simulink model "Power_Grid_Fault_Analysis_2016"  (R2016a)
settings: Solver=FixedStepAuto  SolverMode=SingleTasking  StartTime=0.0  StopTime=0.2  RelTol=1e-3
InitFcn:
  | basekV = 23;
  | baseMVA = 100;
  | 
  | % base impedance
  | baseZ = (basekV)^2/baseMVA;
  | 
  | % nominal frequency
  | freq = 50;
libraries: powerlib x64, powerlib_meascontrol x17
(part 1 of 4)
settings Model: Creator=jywon  LastModifiedBy=md ether
settings DebuggingCC: SFUnexpectedBacktrackingDiag=error  SFNoUnconditionalDefaultTransitionDiag=error
settings SFSimCC: SimUseLocalCustomCode=on
settings RTWCC: RTWUseLocalCustomCode=on
settings GRTTargetCC: TargetLangStandard=C99 (ISO)  GeneratePreprocessorConditionals=Use local settings
settings ConfigComp: CovMetricSettings=dwe  CovHtmlReporting=off  CovSaveCumulativeToWorkspaceVar=off  CovSaveSingleToWorkspaceVar=off  CovExternalEMLEnable=on

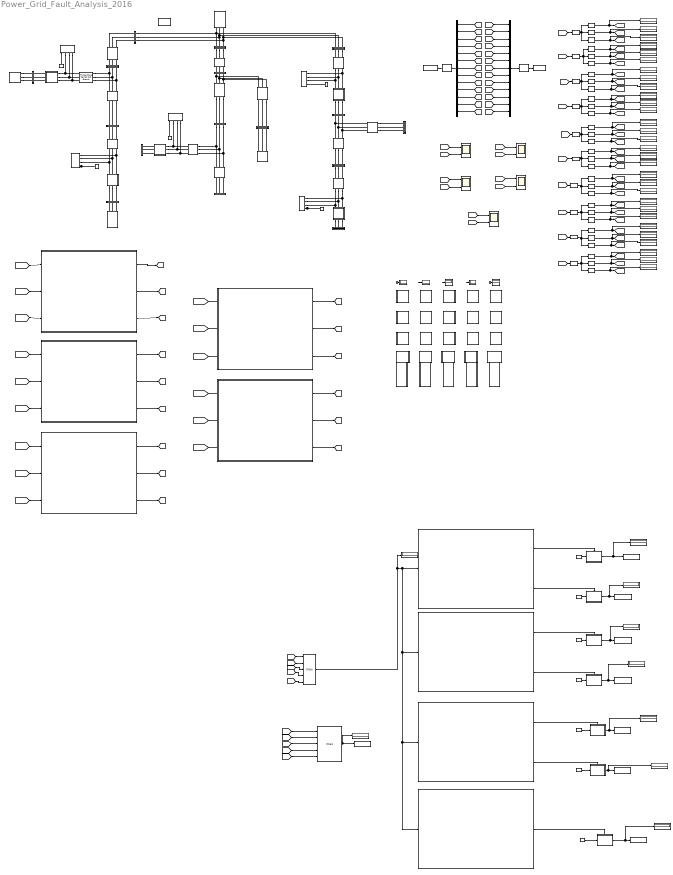
== system Power_Grid_Fault_Analysis_2016 ==
  note: Km S
  note: Fault Phase Detection
  note: Phase Splitter
  note: Zone 1
  note: Zone Voltage and Current
  note: Zone 1
  note: IEEE 16 Bus System
  note: Output Voltage & Current
  note: Zone 2
  note: Zone 5
  note: Zone 4
  note: Zone 3
  note: Zone 1
  note: Zone 2
  note: Zone 3
  note: Zone 4
  note: Zone 5
  note: Zone 2
  note: Zone 3
  note: Zone 4
  note: Zone 5
  note: Km WS
  note: Km S
  note: Km E
  note: Km SE
  Branch1-4 : powerlib/Elements/Three-Phase Series RLC Branch  LConnTagsString=A|B|C  RConnTagsString=A|B|C  BranchType=RL  Resistance=0.075*baseZ  Inductance=(0.1*baseZ)/(2*pi*freq)  Capacitance=1e-6  Measurements=None
  Branch13-14 : powerlib/Elements/Three-Phase Series RLC Branch  LConnTagsString=A|B|C  RConnTagsString=A|B|C  BranchType=RL  Resistance=0.09*baseZ  Inductance=(0.12*baseZ)/(2*pi*freq)  Capacitance=1e-6  Measurements=None
  Branch13-15 : powerlib/Elements/Three-Phase Series RLC Branch  LConnTagsString=A|B|C  RConnTagsString=A|B|C  BranchType=RL  Resistance=0.08*baseZ  Inductance=(0.11*baseZ)/(2*pi*freq)  Capacitance=1e-6  Measurements=None
  Branch15-16 : powerlib/Elements/Three-Phase Series RLC Branch  LConnTagsString=A|B|C  RConnTagsString=A|B|C  BranchType=RL  Resistance=0.04*baseZ  Inductance=(0.04*baseZ)/(2*pi*freq)  Capacitance=1e-6  Measurements=None
  Branch2-8 : powerlib/Elements/Three-Phase Series RLC Branch  LConnTagsString=A|B|C  RConnTagsString=A|B|C  BranchType=RL  Resistance=0.11*baseZ  Inductance=(0.11*baseZ)/(2*pi*freq)  Capacitance=1e-6  Measurements=None
  Branch3-13 : powerlib/Elements/Three-Phase Series RLC Branch  LConnTagsString=A|B|C  RConnTagsString=A|B|C  BranchType=RL  Resistance=0.11*baseZ  Inductance=(0.11*baseZ)/(2*pi*freq)  Capacitance=1e-6  Measurements=None
  Branch4-5 : powerlib/Elements/Three-Phase Series RLC Branch  LConnTagsString=A|B|C  RConnTagsString=A|B|C  BranchType=RL  Resistance=0.08*baseZ  Inductance=(0.11*baseZ)/(2*pi*freq)  Capacitance=1e-6  Measurements=None
  Branch4-6 : powerlib/Elements/Three-Phase Series RLC Branch  LConnTagsString=A|B|C  RConnTagsString=A|B|C  BranchType=RL  Resistance=0.09*baseZ  Inductance=(0.18*baseZ)/(2*pi*freq)  Capacitance=1e-6  Measurements=None
  Branch6-7 : powerlib/Elements/Three-Phase Series RLC Branch  LConnTagsString=A|B|C  RConnTagsString=A|B|C  BranchType=RL  Resistance=0.04  Inductance=(0.04*baseZ)/(2*pi*freq)  Capacitance=1e-6  Measurements=None
  Branch8-10 : powerlib/Elements/Three-Phase Series RLC Branch  LConnTagsString=A|B|C  RConnTagsString=A|B|C  BranchType=RL  Resistance=0.11*baseZ  Inductance=(0.11*baseZ)/(2*pi*freq)  Capacitance=1e-6  Measurements=None
  Branch8-9 : powerlib/Elements/Three-Phase Series RLC Branch  LConnTagsString=A|B|C  RConnTagsString=A|B|C  BranchType=RL  Resistance=0.08*baseZ  Inductance=(0.11*baseZ)/(2*pi*freq)  Capacitance=1e-6  Measurements=None
  Branch9-11 : powerlib/Elements/Three-Phase Series RLC Branch  LConnTagsString=A|B|C  RConnTagsString=A|B|C  BranchType=RL  Resistance=0.11*baseZ  Inductance=(0.11*baseZ)/(2*pi*freq)  Capacitance=1e-6  Measurements=None
  Branch9-12 : powerlib/Elements/Three-Phase Series RLC Branch  LConnTagsString=A|B|C  RConnTagsString=A|B|C  BranchType=RL  Resistance=0.08*baseZ  Inductance=(0.11*baseZ)/(2*pi*freq)  Capacitance=1e-6  Measurements=None
  Bus_1 : Subsystem
  Bus_10 : Subsystem
  Bus_11 : Subsystem
  Bus_12 : Subsystem
  Bus_13 : Subsystem
  Bus_14 : Subsystem
  Bus_15 : Subsystem
  Bus_16 : Subsystem
  Bus_2 : Subsystem
  Bus_3 : Subsystem
  Bus_4 : Subsystem
  Bus_5 : Subsystem
  Bus_6 : Subsystem
  Bus_7 : Subsystem
  Bus_8 : Subsystem
  Bus_9 : Subsystem
  Constant{,1..2,4} (4 alike) : Constant  Value=0
  Constant10 : Constant  Value=5
  Constant11 : Constant  Value=7
  Constant3 : Constant
  Constant5 : Constant  Value=2
  Constant6 : Constant  Value=4
  Constant7 : Constant  Value=3
  Constant8 : Constant
  Constant9 : Constant  Value=6
  Display{,1..43} (44 alike) : Display
      Display settings: Decimation=2
      Display1 settings: Decimation=2
      Display10 settings: Decimation=2
      Display11 settings: Decimation=2
      Display12 settings: Decimation=2
      Display13 settings: Decimation=2
      Display14 settings: Decimation=2
      Display15 settings: Decimation=2
      Display16 settings: Decimation=2
      Display17 settings: Decimation=2
      Display18 settings: Decimation=2
      Display19 settings: Decimation=2
      Display2 settings: Decimation=2
      Display20 settings: Decimation=2
      Display21 settings: Decimation=2
      Display22 settings: Decimation=2
      Display23 settings: Decimation=2
      Display24 settings: Decimation=2
      Display25 settings: Decimation=2
      Display26 settings: Decimation=2
      Display27 settings: Decimation=2
      Display28 settings: Decimation=2
      Display29 settings: Decimation=2
      Display3 settings: Decimation=2
      Display4 settings: Decimation=2
      Display5 settings: Decimation=2
      Display6 settings: Decimation=2
      Display7 settings: Decimation=2
      Display8 settings: Decimation=2
      Display9 settings: Decimation=2
  For Zone 1 : Subsystem
  For Zone 2 : Subsystem
  For Zone 3 : Subsystem
  For Zone 4 : Subsystem
  For Zone 5 : Subsystem
  If : If  IfExpression=u1==1|u1==8|u1==15|u1==22|u1==29  ElseIfExpressions=u1==2|u1==9|u1==16|u1==23|u1==30  ShowElse=off
  If Action Subsystem : Subsystem  TreatAsAtomicUnit=on
  If Action Subsystem1 : Subsystem  TreatAsAtomicUnit=on
  If Action Subsystem2 : Subsystem  TreatAsAtomicUnit=on
  If Action Subsystem3 : Subsystem  TreatAsAtomicUnit=on
  If Action Subsystem4 : Subsystem  TreatAsAtomicUnit=on
  If Action Subsystem5 : Subsystem  TreatAsAtomicUnit=on
  If Action Subsystem6 : Subsystem  TreatAsAtomicUnit=on
  If1 : If  IfExpression=u1==3|u1==10|u1==17|u1==24|u1==31  ElseIfExpressions=u1==4|u1==11|u1==18|u1==25|u1==32  ShowElse=off
  If2 : If  IfExpression=u1==5|u1==12|u1==19|u1==26|u1==33  ElseIfExpressions=u1==6|u1==13|u1==20|u1==27|u1==34  ShowElse=off
  If3 : If  IfExpression=u1==7|u1==14|u1==21|u1==28|u1==35  ShowElse=off
  Incoming1 : powerlib/Electrical Sources/Three-Phase Source  InternalConnection=Yg  VoltagePhases=off  Voltage=basekV*1e3  PhaseAngle=0  Voltage_phases=[25e3 25e3 25e3]/sqrt(3)  PhaseAngles_phases=[0 -120 +120]  Frequency=freq  NonIdealSource=off  SpecifyImpedance=on  Resistance=0.8929  Inductance=16.58e-3  ShortCircuitLevel=438.555e6  BaseVoltage=12.66e3  XRratio=7  BusType=swing  Pref=0  Qref=0  Prefabc=[10e3, 10e3, 10e3]  Qrefabc=[0, 0, 0]  Qmin=-inf  Qmax=inf
  Lamp1 : Subsystem  DialogController=hmiCreateDDGDialog  IsWebBlock=on  mask(MWDashboardBlock){webBlockId=468f77b7-8d3f-43ba-abb4-7f9de16ce9e1, webBlockType=lamp, ShowInLibBrowser=on, ShowInitialText=on, HMISrcModelName=Power_Grid_Fault_Analysis_2016}
      mask prompts: webBlockId "WebBlock Id"; webBlockType "WebBlock Type"; HMISrcModelName "Source Model"
      mask help: Display a color that reflects an input value.
      mask Help: helpview([docroot '/mapfiles/simulink.map'], 'hmi_lamp')
      mask Display:
      | if strcmp(get_param(bdroot(gcb),'BlockDiagramType'),'library')
      |  image([(matlabroot) '/toolbox/simulink/hmi/icons/Lamp.png'])
      | end
  Lamp10 : Subsystem  DialogController=hmiCreateDDGDialog  IsWebBlock=on  mask(MWDashboardBlock){webBlockId=47d835ee-9e52-457b-b3a4-dabcf9efd005, webBlockType=lamp, ShowInLibBrowser=on, ShowInitialText=on, HMISrcModelName=Power_Grid_Fault_Analysis_2016}
      mask prompts: webBlockId "WebBlock Id"; webBlockType "WebBlock Type"; HMISrcModelName "Source Model"
      mask help: Display a color that reflects an input value.
      mask Help: helpview([docroot '/mapfiles/simulink.map'], 'hmi_lamp')
      mask Display:
      | if strcmp(get_param(bdroot(gcb),'BlockDiagramType'),'library')
      |  image([(matlabroot) '/toolbox/simulink/hmi/icons/Lamp.png'])
      | end
  Lamp11 : Subsystem  DialogController=hmiCreateDDGDialog  IsWebBlock=on  mask(MWDashboardBlock){webBlockId=f8b1e46b-6cbe-4fd8-a06e-1cc90b8c3338, webBlockType=lamp, ShowInLibBrowser=on, ShowInitialText=on, HMISrcModelName=Power_Grid_Fault_Analysis_2016}
      mask prompts: webBlockId "WebBlock Id"; webBlockType "WebBlock Type"; HMISrcModelName "Source Model"
      mask help: Display a color that reflects an input value.
      mask Help: helpview([docroot '/mapfiles/simulink.map'], 'hmi_lamp')
      mask Display:
      | if strcmp(get_param(bdroot(gcb),'BlockDiagramType'),'library')
      |  image([(matlabroot) '/toolbox/simulink/hmi/icons/Lamp.png'])
      | end
  Lamp12 : Subsystem  DialogController=hmiCreateDDGDialog  IsWebBlock=on  mask(MWDashboardBlock){webBlockId=2111019f-f01e-48a9-874b-3a281ad1a610, webBlockType=lamp, ShowInLibBrowser=on, ShowInitialText=on, HMISrcModelName=Power_Grid_Fault_Analysis_2016}
      mask prompts: webBlockId "WebBlock Id"; webBlockType "WebBlock Type"; HMISrcModelName "Source Model"
      mask help: Display a color that reflects an input value.
      mask Help: helpview([docroot '/mapfiles/simulink.map'], 'hmi_lamp')
      mask Display:
      | if strcmp(get_param(bdroot(gcb),'BlockDiagramType'),'library')
      |  image([(matlabroot) '/toolbox/simulink/hmi/icons/Lamp.png'])
      | end
  Lamp14 : Subsystem  DialogController=hmiCreateDDGDialog  IsWebBlock=on  mask(MWDashboardBlock){webBlockId=0497d169-c07f-488b-b667-ee60b9bfb21c, webBlockType=lamp, ShowInLibBrowser=on, ShowInitialText=on, HMISrcModelName=Power_Grid_Fault_Analysis_2016}
      mask prompts: webBlockId "WebBlock Id"; webBlockType "WebBlock Type"; HMISrcModelName "Source Model"
      mask help: Display a color that reflects an input value.
      mask Help: helpview([docroot '/mapfiles/simulink.map'], 'hmi_lamp')
      mask Display:
      | if strcmp(get_param(bdroot(gcb),'BlockDiagramType'),'library')
      |  image([(matlabroot) '/toolbox/simulink/hmi/icons/Lamp.png'])
      | end
  Lamp15 : Subsystem  DialogController=hmiCreateDDGDialog  IsWebBlock=on  mask(MWDashboardBlock){webBlockId=37fb807e-8b4a-4eb5-8cd1-eaf9de247767, webBlockType=lamp, ShowInLibBrowser=on, ShowInitialText=on, HMISrcModelName=Power_Grid_Fault_Analysis_2016}
      mask prompts: webBlockId "WebBlock Id"; webBlockType "WebBlock Type"; HMISrcModelName "Source Model"
      mask help: Display a color that reflects an input value.
      mask Help: helpview([docroot '/mapfiles/simulink.map'], 'hmi_lamp')
      mask Display:
      | if strcmp(get_param(bdroot(gcb),'BlockDiagramType'),'library')
      |  image([(matlabroot) '/toolbox/simulink/hmi/icons/Lamp.png'])
      | end
  Lamp16 : Subsystem  DialogController=hmiCreateDDGDialog  IsWebBlock=on  mask(MWDashboardBlock){webBlockId=dff293cc-569e-47d8-a4fe-e96dd9d4666d, webBlockType=lamp, ShowInLibBrowser=on, ShowInitialText=on, HMISrcModelName=Power_Grid_Fault_Analysis_2016}
      mask prompts: webBlockId "WebBlock Id"; webBlockType "WebBlock Type"; HMISrcModelName "Source Model"
      mask help: Display a color that reflects an input value.
      mask Help: helpview([docroot '/mapfiles/simulink.map'], 'hmi_lamp')
      mask Display:
      | if strcmp(get_param(bdroot(gcb),'BlockDiagramType'),'library')
      |  image([(matlabroot) '/toolbox/simulink/hmi/icons/Lamp.png'])
      | end
  Lamp18 : Subsystem  DialogController=hmiCreateDDGDialog  IsWebBlock=on  mask(MWDashboardBlock){webBlockId=13b1519a-e014-4802-8a4a-79357282a9e7, webBlockType=lamp, ShowInLibBrowser=on, ShowInitialText=on, HMISrcModelName=Power_Grid_Fault_Analysis_2016}
      mask prompts: webBlockId "WebBlock Id"; webBlockType "WebBlock Type"; HMISrcModelName "Source Model"
      mask help: Display a color that reflects an input value.
      mask Help: helpview([docroot '/mapfiles/simulink.map'], 'hmi_lamp')
      mask Display:
      | if strcmp(get_param(bdroot(gcb),'BlockDiagramType'),'library')
      |  image([(matlabroot) '/toolbox/simulink/hmi/icons/Lamp.png'])
      | end
  Lamp19 : Subsystem  DialogController=hmiCreateDDGDialog  IsWebBlock=on  mask(MWDashboardBlock){webBlockId=26516c08-3b96-4d03-8fdb-bfe990d7f45b, webBlockType=lamp, ShowInLibBrowser=on, ShowInitialText=on, HMISrcModelName=Power_Grid_Fault_Analysis_2016}
      mask prompts: webBlockId "WebBlock Id"; webBlockType "WebBlock Type"; HMISrcModelName "Source Model"
      mask help: Display a color that reflects an input value.
      mask Help: helpview([docroot '/mapfiles/simulink.map'], 'hmi_lamp')
      mask Display:
      | if strcmp(get_param(bdroot(gcb),'BlockDiagramType'),'library')
      |  image([(matlabroot) '/toolbox/simulink/hmi/icons/Lamp.png'])
      | end
  Lamp2 : Subsystem  DialogController=hmiCreateDDGDialog  IsWebBlock=on  mask(MWDashboardBlock){webBlockId=3d3c35ee-dc2a-417a-bf5a-5478148348c2, webBlockType=lamp, ShowInLibBrowser=on, ShowInitialText=on, HMISrcModelName=Power_Grid_Fault_Analysis_2016}
      mask prompts: webBlockId "WebBlock Id"; webBlockType "WebBlock Type"; HMISrcModelName "Source Model"
      mask help: Display a color that reflects an input value.
      mask Help: helpview([docroot '/mapfiles/simulink.map'], 'hmi_lamp')
      mask Display:
      | if strcmp(get_param(bdroot(gcb),'BlockDiagramType'),'library')
      |  image([(matlabroot) '/toolbox/simulink/hmi/icons/Lamp.png'])
      | end
  Lamp20 : Subsystem  DialogController=hmiCreateDDGDialog  IsWebBlock=on  mask(MWDashboardBlock){webBlockId=6f7fce04-8c20-4fba-bd33-a90a1905ab0b, webBlockType=lamp, ShowInLibBrowser=on, ShowInitialText=on, HMISrcModelName=Power_Grid_Fault_Analysis_2016}
      mask prompts: webBlockId "WebBlock Id"; webBlockType "WebBlock Type"; HMISrcModelName "Source Model"
      mask help: Display a color that reflects an input value.
      mask Help: helpview([docroot '/mapfiles/simulink.map'], 'hmi_lamp')
      mask Display:
      | if strcmp(get_param(bdroot(gcb),'BlockDiagramType'),'library')
      |  image([(matlabroot) '/toolbox/simulink/hmi/icons/Lamp.png'])
      | end
  Lamp21 : Subsystem  DialogController=hmiCreateDDGDialog  IsWebBlock=on  mask(MWDashboardBlock){webBlockId=c64cc1d0-1ee1-41b0-b1ef-29387c8c4faf, webBlockType=lamp, ShowInLibBrowser=on, ShowInitialText=on, HMISrcModelName=Power_Grid_Fault_Analysis_2016}
      mask prompts: webBlockId "WebBlock Id"; webBlockType "WebBlock Type"; HMISrcModelName "Source Model"
      mask help: Display a color that reflects an input value.
      mask Help: helpview([docroot '/mapfiles/simulink.map'], 'hmi_lamp')
      mask Display:
      | if strcmp(get_param(bdroot(gcb),'BlockDiagramType'),'library')
      |  image([(matlabroot) '/toolbox/simulink/hmi/icons/Lamp.png'])
      | end
  Lamp22 : Subsystem  DialogController=hmiCreateDDGDialog  IsWebBlock=on  mask(MWDashboardBlock){webBlockId=845159ea-2f47-481f-a3ef-47166ce66799, webBlockType=lamp, ShowInLibBrowser=on, ShowInitialText=on, HMISrcModelName=Power_Grid_Fault_Analysis_2016}
      mask prompts: webBlockId "WebBlock Id"; webBlockType "WebBlock Type"; HMISrcModelName "Source Model"
      mask help: Display a color that reflects an input value.
      mask Help: helpview([docroot '/mapfiles/simulink.map'], 'hmi_lamp')
      mask Display:
      | if strcmp(get_param(bdroot(gcb),'BlockDiagramType'),'library')
      |  image([(matlabroot) '/toolbox/simulink/hmi/icons/Lamp.png'])
      | end
  Lamp23 : Subsystem  DialogController=hmiCreateDDGDialog  IsWebBlock=on  mask(MWDashboardBlock){webBlockId=af2698c2-590e-4ed0-a645-40a46a76e42b, webBlockType=lamp, ShowInLibBrowser=on, ShowInitialText=on, HMISrcModelName=Power_Grid_Fault_Analysis_2016}
      mask prompts: webBlockId "WebBlock Id"; webBlockType "WebBlock Type"; HMISrcModelName "Source Model"
      mask help: Display a color that reflects an input value.
      mask Help: helpview([docroot '/mapfiles/simulink.map'], 'hmi_lamp')
      mask Display:
      | if strcmp(get_param(bdroot(gcb),'BlockDiagramType'),'library')
      |  image([(matlabroot) '/toolbox/simulink/hmi/icons/Lamp.png'])
      | end
  Lamp3 : Subsystem  DialogController=hmiCreateDDGDialog  IsWebBlock=on  mask(MWDashboardBlock){webBlockId=b3a08374-8d73-4b38-9446-1522d8dad8a0, webBlockType=lamp, ShowInLibBrowser=on, ShowInitialText=on, HMISrcModelName=Power_Grid_Fault_Analysis_2016}
      mask prompts: webBlockId "WebBlock Id"; webBlockType "WebBlock Type"; HMISrcModelName "Source Model"
      mask help: Display a color that reflects an input value.
      mask Help: helpview([docroot '/mapfiles/simulink.map'], 'hmi_lamp')
      mask Display:
      | if strcmp(get_param(bdroot(gcb),'BlockDiagramType'),'library')
      |  image([(matlabroot) '/toolbox/simulink/hmi/icons/Lamp.png'])
      | end
  Lamp4 : Subsystem  DialogController=hmiCreateDDGDialog  IsWebBlock=on  mask(MWDashboardBlock){webBlockId=b5af589e-626e-4b25-93a4-676fcf5d279b, webBlockType=lamp, ShowInLibBrowser=on, ShowInitialText=on, HMISrcModelName=Power_Grid_Fault_Analysis_2016}
      mask prompts: webBlockId "WebBlock Id"; webBlockType "WebBlock Type"; HMISrcModelName "Source Model"
      mask help: Display a color that reflects an input value.
      mask Help: helpview([docroot '/mapfiles/simulink.map'], 'hmi_lamp')
      mask Display:
      | if strcmp(get_param(bdroot(gcb),'BlockDiagramType'),'library')
      |  image([(matlabroot) '/toolbox/simulink/hmi/icons/Lamp.png'])
      | end
  Lamp5 : Subsystem  DialogController=hmiCreateDDGDialog  IsWebBlock=on  mask(MWDashboardBlock){webBlockId=8c5f1737-98a7-4483-befe-b85a709fdb78, webBlockType=lamp, ShowInLibBrowser=on, ShowInitialText=on, HMISrcModelName=Power_Grid_Fault_Analysis_2016}
      mask prompts: webBlockId "WebBlock Id"; webBlockType "WebBlock Type"; HMISrcModelName "Source Model"
      mask help: Display a color that reflects an input value.
      mask Help: helpview([docroot '/mapfiles/simulink.map'], 'hmi_lamp')
      mask Display:
      | if strcmp(get_param(bdroot(gcb),'BlockDiagramType'),'library')
      |  image([(matlabroot) '/toolbox/simulink/hmi/icons/Lamp.png'])
      | end
  Lamp6 : Subsystem  DialogController=hmiCreateDDGDialog  IsWebBlock=on  mask(MWDashboardBlock){webBlockId=54263707-eb2a-444c-8d6c-36b23799e939, webBlockType=lamp, ShowInLibBrowser=on, ShowInitialText=on, HMISrcModelName=Power_Grid_Fault_Analysis_2016}
      mask prompts: webBlockId "WebBlock Id"; webBlockType "WebBlock Type"; HMISrcModelName "Source Model"
      mask help: Display a color that reflects an input value.
      mask Help: helpview([docroot '/mapfiles/simulink.map'], 'hmi_lamp')
      mask Display:
      | if strcmp(get_param(bdroot(gcb),'BlockDiagramType'),'library')
      |  image([(matlabroot) '/toolbox/simulink/hmi/icons/Lamp.png'])
      | end
  Lamp7 : Subsystem  DialogController=hmiCreateDDGDialog  IsWebBlock=on  mask(MWDashboardBlock){webBlockId=44ba34c8-8d6e-4af3-8262-8e210390e885, webBlockType=lamp, ShowInLibBrowser=on, ShowInitialText=on, HMISrcModelName=Power_Grid_Fault_Analysis_2016}
      mask prompts: webBlockId "WebBlock Id"; webBlockType "WebBlock Type"; HMISrcModelName "Source Model"
      mask help: Display a color that reflects an input value.
      mask Help: helpview([docroot '/mapfiles/simulink.map'], 'hmi_lamp')
      mask Display:
      | if strcmp(get_param(bdroot(gcb),'BlockDiagramType'),'library')
      |  image([(matlabroot) '/toolbox/simulink/hmi/icons/Lamp.png'])
      | end
  Lamp9 : Subsystem  DialogController=hmiCreateDDGDialog  IsWebBlock=on  mask(MWDashboardBlock){webBlockId=ca856779-7c2c-42aa-8051-6cc6fb4e4d11, webBlockType=lamp, ShowInLibBrowser=on, ShowInitialText=on, HMISrcModelName=Power_Grid_Fault_Analysis_2016}
      mask prompts: webBlockId "WebBlock Id"; webBlockType "WebBlock Type"; HMISrcModelName "Source Model"
      mask help: Display a color that reflects an input value.
      mask Help: helpview([docroot '/mapfiles/simulink.map'], 'hmi_lamp')
      mask Display:
      | if strcmp(get_param(bdroot(gcb),'BlockDiagramType'),'library')
      |  image([(matlabroot) '/toolbox/simulink/hmi/icons/Lamp.png'])
      | end
  Max : MinMax  Function=max  Inputs=5
  Max1 : MinMax  Function=max  Inputs=5
  Mux : Mux  Inputs=13
  Mux1 : Mux  Inputs=13
  RMS{,1..11} (12 alike) : powerlib_meascontrol/Measurements/RMS  TrueRMS=on  Freq=freq  RMSInit=0  Ts=0
  "Relay " : Subsystem
  Relay 1 : Subsystem
  Relay 2 : Subsystem
  Relay 3 : Subsystem
  Relay 4 : Subsystem
  Scope{,1..4} (5 alike) : Scope  NumInputPorts=2
  Selector{,3,6,9,14,17,20,23,26,29} (10 alike) : Selector  InputPortWidth=3  IndexOptions=Index vector (dialog)  Indices=[1]  OutputSizes=1
  Selector{1,4,7,10,12,15,18,21,24,27} (10 alike) : Selector  InputPortWidth=3  IndexOptions=Index vector (dialog)  Indices=[2]  OutputSizes=1
  Selector{2,5,8,11,13,16,19,22,25,28} (10 alike) : Selector  InputPortWidth=3  IndexOptions=Index vector (dialog)  Indices=[3]  OutputSizes=1
  Three-Phase Fault1 : powerlib/Elements/Three-Phase Fault  InitialStates=[0 0 0]  FaultA=on  FaultB=off  FaultC=off  GroundFault=on  SwitchTimes="[1/60  5/60]"  External=on  SwitchStatus=NaN  FaultResistance=0.1  GroundResistance=0.01  SnubberResistance=1e6  SnubberCapacitance=inf  Measurements=None
  Three-Phase Fault2 : powerlib/Elements/Three-Phase Fault  InitialStates=[0 0 0]  FaultA=on  FaultB=on  FaultC=off  GroundFault=on  SwitchTimes="[1/60  5/60]"  External=on  SwitchStatus=NaN  FaultResistance=0.1  GroundResistance=0.01  SnubberResistance=1e6  SnubberCapacitance=inf  Measurements=None
  Three-Phase Fault3 : powerlib/Elements/Three-Phase Fault  InitialStates=[0 0 0]  FaultA=on  FaultB=on  FaultC=on  GroundFault=on  SwitchTimes="[1/60  5/60]"  External=on  SwitchStatus=NaN  FaultResistance=0.1  GroundResistance=0.01  SnubberResistance=1e6  SnubberCapacitance=inf  Measurements=None
  Three-Phase Fault4 : powerlib/Elements/Three-Phase Fault  InitialStates=[0 0 0]  FaultA=on  FaultB=off  FaultC=off  GroundFault=on  SwitchTimes="[1/60  5/60]"  External=on  SwitchStatus=NaN  FaultResistance=0.1  GroundResistance=0.01  SnubberResistance=1e6  SnubberCapacitance=inf  Measurements=None
  Three-Phase Fault5 : powerlib/Elements/Three-Phase Fault  InitialStates=[0 0 0]  FaultA=on  FaultB=off  FaultC=off  GroundFault=on  SwitchTimes="[1/60  5/60]"  External=on  SwitchStatus=NaN  FaultResistance=0.1  GroundResistance=0.01  SnubberResistance=1e6  SnubberCapacitance=inf  Measurements=None
  Tieline10-14 : powerlib/Elements/Three-Phase Series RLC Branch  LConnTagsString=A|B|C  RConnTagsString=A|B|C  BranchType=RL  Resistance=0.04*baseZ  Inductance=(0.04*baseZ)/(2*pi*freq)  Capacitance=1e-6  Measurements=None
  Tieline5-11 : powerlib/Elements/Three-Phase Series RLC Branch  LConnTagsString=A|B|C  RConnTagsString=A|B|C  BranchType=RL  Resistance=0.04*baseZ  Inductance=(0.04*baseZ)/(2*pi*freq)  Capacitance=1e-6  Measurements=None
  Tieline7-16 : powerlib/Elements/Three-Phase Series RLC Branch  LConnTagsString=A|B|C  RConnTagsString=A|B|C  BranchType=RL  Resistance=0.09*baseZ  Inductance=(0.12*baseZ)/(2*pi*freq)  Capacitance=1e-6  Measurements=None
  To Workspace : ToWorkspace  VariableName=simOutputV  SaveFormat=Timeseries  SampleTime=-1
  To Workspace1 : ToWorkspace  VariableName=simOutputI  SaveFormat=Timeseries  SampleTime=-1
  To Workspace2 : ToWorkspace  VariableName=Distance  SaveFormat=Timeseries  SampleTime=-1
  To Workspace3 : ToWorkspace  VariableName=A  SaveFormat=Timeseries  SampleTime=-1
  To Workspace4 : ToWorkspace  VariableName=B  SaveFormat=Timeseries  SampleTime=-1
  To Workspace5 : ToWorkspace  VariableName=C  SaveFormat=Timeseries  SampleTime=-1
  To Workspace6 : ToWorkspace  VariableName=AB  SaveFormat=Timeseries  SampleTime=-1
  To Workspace7 : ToWorkspace  VariableName=BC  SaveFormat=Timeseries  SampleTime=-1
  To Workspace8 : ToWorkspace  VariableName=CA  SaveFormat=Timeseries  SampleTime=-1
  To Workspace9 : ToWorkspace  VariableName=ABC  SaveFormat=Timeseries  SampleTime=-1
  Toggle Switch : Subsystem  DialogController=hmiCreateDDGDialog  IsWebBlock=on  mask(MWDashboardBlock){webBlockId=0d8ce81f-dbe4-4348-a7f3-529ab13bc594, webBlockType=toggleswitch, ShowInLibBrowser=on, ShowInitialText=on, HMISrcModelName=Power_Grid_Fault_Analysis_2016}
      mask prompts: webBlockId "WebBlock Id"; webBlockType "WebBlock Type"; HMISrcModelName "Source Model"
      mask help: Set on/off value to tune parameters or variables.
      mask Help: helpview([docroot '/mapfiles/simulink.map'], 'hmi_switch')
      mask Display:
      | if strcmp(get_param(bdroot(gcb),'BlockDiagramType'),'library')
      |  image([(matlabroot) '/toolbox/simulink/hmi/icons/ToggleSwitch.png'])
      | end
  Toggle Switch1 : Subsystem  DialogController=hmiCreateDDGDialog  IsWebBlock=on  mask(MWDashboardBlock){webBlockId=5b9374ce-f1d7-4d86-b5a1-51c8e36ab682, webBlockType=toggleswitch, ShowInLibBrowser=on, ShowInitialText=on, HMISrcModelName=Power_Grid_Fault_Analysis_2016}
      mask prompts: webBlockId "WebBlock Id"; webBlockType "WebBlock Type"; HMISrcModelName "Source Model"
      mask help: Set on/off value to tune parameters or variables.
      mask Help: helpview([docroot '/mapfiles/simulink.map'], 'hmi_switch')
      mask Display:
      | if strcmp(get_param(bdroot(gcb),'BlockDiagramType'),'library')
      |  image([(matlabroot) '/toolbox/simulink/hmi/icons/ToggleSwitch.png'])
      | end
  Toggle Switch2 : Subsystem  DialogController=hmiCreateDDGDialog  IsWebBlock=on  mask(MWDashboardBlock){webBlockId=a5a22a72-9f9a-45fa-8f0f-c647fe18b1da, webBlockType=toggleswitch, ShowInLibBrowser=on, ShowInitialText=on, HMISrcModelName=Power_Grid_Fault_Analysis_2016}
      mask prompts: webBlockId "WebBlock Id"; webBlockType "WebBlock Type"; HMISrcModelName "Source Model"
      mask help: Set on/off value to tune parameters or variables.
      mask Help: helpview([docroot '/mapfiles/simulink.map'], 'hmi_switch')
      mask Display:
      | if strcmp(get_param(bdroot(gcb),'BlockDiagramType'),'library')
      |  image([(matlabroot) '/toolbox/simulink/hmi/icons/ToggleSwitch.png'])
      | end
  Toggle Switch3 : Subsystem  DialogController=hmiCreateDDGDialog  IsWebBlock=on  mask(MWDashboardBlock){webBlockId=58ae28e7-e799-496d-825d-186d552e1de1, webBlockType=toggleswitch, ShowInLibBrowser=on, ShowInitialText=on, HMISrcModelName=Power_Grid_Fault_Analysis_2016}
      mask prompts: webBlockId "WebBlock Id"; webBlockType "WebBlock Type"; HMISrcModelName "Source Model"
      mask help: Set on/off value to tune parameters or variables.
      mask Help: helpview([docroot '/mapfiles/simulink.map'], 'hmi_switch')
      mask Display:
      | if strcmp(get_param(bdroot(gcb),'BlockDiagramType'),'library')
      |  image([(matlabroot) '/toolbox/simulink/hmi/icons/ToggleSwitch.png'])
      | end
  Toggle Switch4 : Subsystem  DialogController=hmiCreateDDGDialog  IsWebBlock=on  mask(MWDashboardBlock){webBlockId=0e496b9f-e035-48d9-ae06-0f0cf0e7b1be, webBlockType=toggleswitch, ShowInLibBrowser=on, ShowInitialText=on, HMISrcModelName=Power_Grid_Fault_Analysis_2016}
      mask prompts: webBlockId "WebBlock Id"; webBlockType "WebBlock Type"; HMISrcModelName "Source Model"
      mask help: Set on/off value to tune parameters or variables.
      mask Help: helpview([docroot '/mapfiles/simulink.map'], 'hmi_switch')
      mask Display:
      | if strcmp(get_param(bdroot(gcb),'BlockDiagramType'),'library')
      |  image([(matlabroot) '/toolbox/simulink/hmi/icons/ToggleSwitch.png'])
      | end
  powergui1 : powerlib/powergui  Priority=1  SimulationMode=Discrete  SampleTime=50e-6  frequency=60  Iterations=50  frequencyindice=50  Pbase=100e6  ErrMax=0.0001  UnitsV=kV  UnitsW=MW  buscounter=0  FunctionMessages=off  echomessages=off  EnableUseOfTLC=off  CurrentSourceSwitches=off  DisableSnubberDevices=off  DisableRonSwitches=off  DisableVfSwitches=off  DisplayEquations=off  AutomaticDiscreteSolvers=off  SolverType=Tustin/Backward Euler (TBE)  Interpol=off  ExternalGateDelay=off  methode=off  Ts=100  x0status=blocks  SPID=off  SwTol=0  HookPort=off  NonlinearTolerance=0  nMaxIteration=15  ContinueOnMaxIteration=off  RestoreLinks=warning  ResistiveCurrentMeasurement=off  Frange=[0:2:500]  Ylog=off  Xlog=on  ShowGrid=off  save=off  variable=ZData  structure=0  ZoomFFT=off  StartTime=0.0  cycles=1  DisplayStyle=1  fundamental=60  FreqAxis=off  MaxFrequency=1000  frequencyindicesteady=1  RmsSteady=2  display=off
  tag scope: B_2=global, B_5=global
  wires:
  [V13to15] -> Mux/12
  [V6to7] -> Mux/4
  [V2to8] -> Mux/5
  [V13to14] -> Mux/11
  [V4to6] -> Mux/3
  [V8to9] -> Mux/6
  [V4to5] -> Mux/2
  [V15to16] -> Mux/13
  Mux/1 -> RMS/1
  [V9to11] -> Mux/8
  [V1to4] -> Mux/1
  [V8to10] -> Mux/7
  [V3to13] -> Mux/10
  RMS1/1 -> To Workspace1/1
  RMS/1 -> To Workspace/1
  [V9to12] -> Mux/9
  [I8to9] -> Mux1/6
  [I13to14] -> Mux1/11
  [I6to7] -> Mux1/4
  [I2to8] -> Mux1/5
  [I1to4] -> Mux1/1
  [I4to5] -> Mux1/2
  [I13to15] -> Mux1/12
  [I9to12] -> Mux1/9
  [I3to13] -> Mux1/10
  [I15to16] -> Mux1/13
  [I4to6] -> Mux1/3
  [I9to11] -> Mux1/8
  [I8to10] -> Mux1/7
  Mux1/1 -> RMS1/1
  Constant3/1 -> Three-Phase Fault2/1  "Bus 3-13 Fault"
  [V4to5] -> Scope/1
  [I4to5] -> Scope/2
  Constant4/1 -> [B_5], Three-Phase Fault1/1  "Bus 15-16 Fault"
  Constant2/1 -> Three-Phase Fault3/1  "Bus 9-11 Fault"
  Constant1/1 -> [B_2], Three-Phase Fault4/1  "Bus 6-7 Fault"
  Constant/1 -> Three-Phase Fault5/1  "Z1"
  [I6to7] -> Scope1/2
  [V6to7] -> Scope1/1
  [V3to13] -> Scope3/1
  [I3to13] -> Scope3/2
  [I9to11] -> Scope2/2
  [V9to11] -> Scope2/1
  [I15to16] -> Scope4/2
  [V15to16] -> Scope4/1
  RMS3/1 -> Selector2/1, Selector1/1, Selector/1
  [I4to5] -> RMS2/1
  Selector/1 -> Display/1, [Z1_Va]
  Selector1/1 -> Display1/1, [Z1_Vb]
  Selector2/1 -> Display2/1, [Z1_Vc]
  Selector11/1 -> Display11/1, [Z2_Ic]
  Selector10/1 -> Display10/1, [Z2_Ib]
  Selector9/1 -> Display9/1, [Z2_Ia]
  Selector8/1 -> Display8/1, [Z2_Vc]
  Selector7/1 -> Display7/1, [Z2_Vb]
  Selector6/1 -> Display6/1, [Z2_Va]
  RMS5/1 -> Selector9/1, Selector10/1, Selector11/1
  RMS4/1 -> Selector6/1, Selector7/1, Selector8/1
  Selector13/1 -> Display13/1, [Z3_Ic]
  RMS7/1 -> Selector17/1, Selector12/1, Selector13/1
  Selector15/1 -> Display15/1, [Z3_Vb]
  Selector14/1 -> Display14/1, [Z3_Va]
  RMS6/1 -> Selector14/1, Selector15/1, Selector16/1
  Selector17/1 -> Display17/1, [Z3_Ia]
  Selector12/1 -> Display12/1, [Z3_Ib]
  Selector16/1 -> Display16/1, [Z3_Vc]
  Selector22/1 -> Display22/1, [Z4_Vc]
  Selector18/1 -> Display18/1, [Z4_Ib]
  Selector23/1 -> Display23/1, [Z4_Ia]
  RMS8/1 -> Selector20/1, Selector21/1, Selector22/1
  Selector20/1 -> Display20/1, [Z4_Va]
  Selector21/1 -> Display21/1, [Z4_Vb]
  RMS9/1 -> Selector23/1, Selector18/1, Selector19/1
  Selector19/1 -> Display19/1, [Z4_Ic]
  Selector24/1 -> Display24/1, [Z5_Ib]
  Selector28/1 -> Display28/1, [Z5_Vc]
  RMS10/1 -> Selector26/1, Selector27/1, Selector28/1
  Selector29/1 -> Display29/1, [Z5_Ia]
  Selector25/1 -> Display25/1, [Z5_Ic]
  RMS11/1 -> Selector29/1, Selector24/1, Selector25/1
  Selector27/1 -> Display27/1, [Z5_Vb]
  Selector26/1 -> Display26/1, [Z5_Va]
  Selector3/1 -> Display3/1, [Z1_Ia]
  Selector4/1 -> Display4/1, [Z1_Ib]
  Selector5/1 -> Display5/1, [Z1_Ic]
  RMS2/1 -> Selector3/1, Selector5/1, Selector4/1
  [V4to5] -> RMS3/1
  [V6to7] -> RMS4/1
  [I6to7] -> RMS5/1
  [V9to11] -> RMS6/1
  [I9to11] -> RMS7/1
  [V3to13] -> RMS8/1
  [I3to13] -> RMS9/1
  [V15to16] -> RMS10/1
  [I15to16] -> RMS11/1
  [Z1_Ia] -> For Zone 1/1(Phase A)
  [Z1_Ic] -> For Zone 1/3(Phase C)
  [Z1_Ib] -> For Zone 1/2(Phase B)
  For Zone 1/1(Phase a) -> [Z1_Y1]  "A"
  For Zone 1/2(Phase b) -> [Z1_Y2]  "B"
  For Zone 1/3(Phase c) -> [Z1_Y3]  "C"
  [Z2_Ic] -> For Zone 2/3(Phase C)
  For Zone 2/3(Phase c) -> [Z2_Y3]  "C"
  [Z2_Ib] -> For Zone 2/2(Phase B)
  [Z2_Ia] -> For Zone 2/1(Phase A)
  For Zone 2/1(Phase a) -> [Z2_Y1]  "A"
  For Zone 2/2(Phase b) -> [Z2_Y2]  "B"
  For Zone 3/1(Phase a) -> [Z3_Y1]  "A"
  For Zone 3/2(Phase b) -> [Z3_Y2]  "B"
  [Z3_Ib] -> For Zone 3/2(Phase B)
  [Z3_Ia] -> For Zone 3/1(Phase A)
  For Zone 3/3(Phase c) -> [Z3_Y3]  "C"
  [Z3_Ic] -> For Zone 3/3(Phase C)
  For Zone 4/2(Phase b) -> [Z4_Y2]  "B"
  For Zone 4/1(Phase a) -> [Z4_Y1]  "A"
  [Z4_Ia] -> For Zone 4/1(Phase A)
  [Z5_Ib] -> For Zone 5/2(Phase B)
  [Z4_Ic] -> For Zone 4/3(Phase C)
  [Z5_Ia] -> For Zone 5/1(Phase A)
  [Z4_Ib] -> For Zone 4/2(Phase B)
  For Zone 5/2(Phase b) -> [Z5_Y2]  "B"
  For Zone 5/1(Phase a) -> [Z5_Y1]  "A"
  [Z5_Ic] -> For Zone 5/3(Phase C)
  For Zone 5/3(Phase c) -> [Z5_Y3]  "C"
  For Zone 4/3(Phase c) -> [Z4_Y3]  "C"
  [D_Z_5] -> Display30/1
  [D_Z_4] -> Display31/1
  [D_Z_3] -> Display32/1
  [D_Z_2] -> Display33/1
  [D_Z_1] -> Display34/1
  Max/1 -> Display35/1, To Workspace2/1
  [D_Z_1] -> Max/1
  [D_Z_2] -> Max/2
  [D_Z_3] -> Max/3
  [D_Z_4] -> Max/4
  [D_Z_5] -> Max/5
  Constant8/1 -> If Action Subsystem/1(Input)
  If/1 -> If Action Subsystem/Action
  If Action Subsystem1/1(Out1) -> Display38/1, To Workspace4/1
  If/2 -> If Action Subsystem1/Action
  Constant5/1 -> If Action Subsystem1/1(Input)
  Constant6/1 -> If Action Subsystem3/1(Input)
  If1/1 -> If Action Subsystem2/Action
  Constant7/1 -> If Action Subsystem2/1(Input)
  If Action Subsystem3/1(Out1) -> Display40/1, To Workspace6/1
  If1/2 -> If Action Subsystem3/Action
  Constant10/1 -> If Action Subsystem4/1(Input)
  If2/1 -> If Action Subsystem4/Action
  If Action Subsystem4/1(Out1) -> Display41/1, To Workspace7/1
  Constant9/1 -> If Action Subsystem5/1(Input)
  If2/2 -> If Action Subsystem5/Action
  Max1/1 -> If3/1, If2/1, If1/1, If/1, Display37/1
  Constant11/1 -> If Action Subsystem6/1(Input)
  If3/1 -> If Action Subsystem6/Action
  If Action Subsystem6/1(Out1) -> To Workspace9/1, Display43/1
  If Action Subsystem/1(Out1) -> Display36/1, To Workspace3/1
  [F_1_Z] -> Max1/1
  [F_2_Z] -> Max1/2
  [F_3_Z] -> Max1/3
  [F_4_Z] -> Max1/4
  [F_4_Z] -> Max1/5
  If Action Subsystem2/1(Out1) -> Display39/1, To Workspace5/1
  If Action Subsystem5/1(Out1) -> Display42/1, To Workspace8/1
  connections:
  Bus_2/LConn2 -- Incoming1/RConn2 -- Bus_3/LConn2 -- Bus_1/LConn2
  Bus_2/RConn1 -- Branch2-8/LConn1
  Bus_2/LConn1 -- Incoming1/RConn1 -- Bus_1/LConn1 -- Bus_3/LConn1
  Bus_2/RConn3 -- Branch2-8/LConn3
  Bus_2/LConn3 -- Bus_3/LConn3 -- Incoming1/RConn3 -- Bus_1/LConn3
  Bus_2/RConn2 -- Branch2-8/LConn2
  Branch1-4/LConn3 -- Bus_1/RConn3
  Branch1-4/LConn1 -- Bus_1/RConn1
  Bus_3/RConn3 -- Branch3-13/LConn3
  Bus_3/RConn2 -- Branch3-13/LConn2
  Branch3-13/LConn1 -- Bus_3/RConn1
  Bus_4/LConn3 -- Branch1-4/RConn3
  Bus_4/LConn2 -- Branch1-4/RConn2
  Bus_4/LConn1 -- Branch1-4/RConn1
  Branch4-6/LConn3 -- Branch4-5/LConn3 -- Bus_4/RConn3
  Branch4-6/LConn2 -- Branch4-5/LConn2 -- Bus_4/RConn2
  Branch4-6/LConn1 -- Bus_4/RConn1 -- Branch4-5/LConn1
  Bus_6/LConn3 -- Branch4-6/RConn3
  Bus_6/LConn2 -- Branch4-6/RConn2
  Bus_6/LConn1 -- Branch4-6/RConn1
  Branch6-7/LConn3 -- Bus_6/RConn3
  Branch6-7/LConn2 -- Bus_6/RConn2
  Branch6-7/LConn1 -- Bus_6/RConn1
  Bus_8/LConn3 -- Branch2-8/RConn3
  Bus_8/LConn2 -- Branch2-8/RConn2
  Bus_8/LConn1 -- Branch2-8/RConn1
  Bus_8/RConn2 -- Branch8-10/LConn2 -- Branch8-9/LConn2
  Bus_8/RConn1 -- Branch8-10/LConn1 -- Branch8-9/LConn1
  Bus_8/RConn3 -- Branch8-10/LConn3 -- Branch8-9/LConn3
  Branch8-9/RConn1 -- Bus_9/LConn1
  Branch8-9/RConn2 -- Bus_9/LConn2
  Branch8-9/RConn3 -- Bus_9/LConn3
  Bus_9/RConn2 -- Branch9-12/LConn2 -- Branch9-11/LConn2
  Bus_9/RConn1 -- Branch9-12/LConn1 -- Branch9-11/LConn1
  Bus_9/RConn3 -- Branch9-12/LConn3 -- Branch9-11/LConn3
  Bus_12/LConn1 -- Branch9-12/RConn1
  Bus_12/LConn2 -- Branch9-12/RConn2
  Bus_12/LConn3 -- Branch9-12/RConn3
  Bus_10/LConn1 -- Branch8-10/RConn1
  Bus_10/LConn2 -- Branch8-10/RConn2
  Branch8-10/RConn3 -- Bus_10/LConn3
  Branch13-15/LConn3 -- Bus_13/RConn3 -- Branch13-14/LConn3
  Branch13-15/LConn2 -- Bus_13/RConn2 -- Branch13-14/LConn2
  Branch13-15/LConn1 -- Bus_13/RConn1 -- Branch13-14/LConn1
  Branch13-15/RConn1 -- Bus_15/LConn1
  Branch13-15/RConn2 -- Bus_15/LConn2
  Branch13-15/RConn3 -- Bus_15/LConn3
  Branch13-14/RConn3 -- Bus_14/LConn3
  Bus_14/LConn2 -- Branch13-14/RConn2
  Branch13-14/RConn1 -- Bus_14/LConn1
  Branch15-16/LConn3 -- Bus_15/RConn3
  Bus_15/RConn2 -- Branch15-16/LConn2
  Bus_15/RConn1 -- Branch15-16/LConn1
  Tieline5-11/LConn1 -- Bus_5/RConn1
  Tieline5-11/LConn2 -- Bus_5/RConn2
  Tieline5-11/LConn3 -- Bus_5/RConn3
  Tieline10-14/LConn1 -- Bus_10/RConn1
  Tieline10-14/LConn2 -- Bus_10/RConn2
  Tieline10-14/LConn3 -- Bus_10/RConn3
  Tieline7-16/LConn1 -- Bus_7/RConn1
  Tieline7-16/LConn2 -- Bus_7/RConn2
  Tieline7-16/LConn3 -- Bus_7/RConn3
  "Relay "/RConn1 -- Bus_13/LConn1
  "Relay "/RConn2 -- Bus_13/LConn2
  "Relay "/RConn3 -- Bus_13/LConn3
  Three-Phase Fault2/LConn3 -- "Relay "/LConn3 -- Branch3-13/RConn3
  Branch3-13/RConn2 -- "Relay "/LConn2 -- Three-Phase Fault2/LConn2
  Branch3-13/RConn1 -- "Relay "/LConn1 -- Three-Phase Fault2/LConn1
  Branch15-16/RConn1 -- Relay 1/LConn1 -- Three-Phase Fault1/LConn1
  Branch15-16/RConn2 -- Relay 1/LConn2 -- Three-Phase Fault1/LConn2
  Branch15-16/RConn3 -- Relay 1/LConn3 -- Three-Phase Fault1/LConn3
  Relay 1/RConn1 -- Bus_16/LConn1
  Relay 1/RConn2 -- Bus_16/LConn2
  Relay 1/RConn3 -- Bus_16/LConn3
  Relay 2/LConn1 -- Branch9-11/RConn1 -- Three-Phase Fault3/LConn1
  Relay 2/LConn2 -- Branch9-11/RConn2 -- Three-Phase Fault3/LConn2
  Relay 2/LConn3 -- Branch9-11/RConn3 -- Three-Phase Fault3/LConn3
  Relay 2/RConn3 -- Bus_11/LConn3
  Relay 2/RConn2 -- Bus_11/LConn2
  Relay 2/RConn1 -- Bus_11/LConn1
  Relay 3/LConn3 -- Branch6-7/RConn3 -- Three-Phase Fault4/LConn3
  Relay 3/LConn1 -- Branch6-7/RConn1 -- Three-Phase Fault4/LConn1
  Relay 3/LConn2 -- Branch6-7/RConn2 -- Three-Phase Fault4/LConn2
  Relay 3/RConn2 -- Bus_7/LConn2
  Relay 3/RConn1 -- Bus_7/LConn1
  Relay 3/RConn3 -- Bus_7/LConn3
  Relay 4/LConn3 -- Branch4-5/RConn3 -- Three-Phase Fault5/LConn3
  Relay 4/LConn1 -- Branch4-5/RConn1 -- Three-Phase Fault5/LConn1
  Relay 4/LConn2 -- Branch4-5/RConn2 -- Three-Phase Fault5/LConn2
  Relay 4/RConn3 -- Bus_5/LConn3
  Relay 4/RConn2 -- Bus_5/LConn2
  Relay 4/RConn1 -- Bus_5/LConn1
  Bus_1/RConn2 -- Branch1-4/LConn2

== system Power_Grid_Fault_Analysis_2016/Bus_1 ==
  Bus_1 : powerlib/Measurements/Three-Phase V-I Measurement  VoltageMeasurement=phase-to-phase  SetLabelV=off  LabelV=Vabc  Vpu=off  VpuLL=off  CurrentMeasurement=yes  SetLabelI=off  LabelI=Iabc  Ipu=off  Pbase=100e6  Vbase=500e3  OutputType=Complex  PhasorSimulation=off  PSBequivalent=0
  Terminator : Terminator
  Terminator1 : Terminator
  InPhaseA : PMIOPort  Side=Left
  InPhaseB : PMIOPort  Port=2  Side=Left
  InPhaseC : PMIOPort  Port=3  Side=Left
  OutPhaseA : PMIOPort  Port=4  Side=Right
  OutPhaseB : PMIOPort  Port=5  Side=Right
  OutPhaseC : PMIOPort  Port=6  Side=Right
  wires:
  Bus_1/1 -> Terminator/1
  Bus_1/2 -> Terminator1/1
  connections:
  OutPhaseA/RConn1 -- Bus_1/RConn1
  OutPhaseB/RConn1 -- Bus_1/RConn2
  OutPhaseC/RConn1 -- Bus_1/RConn3
  InPhaseA/RConn1 -- Bus_1/LConn1
  InPhaseB/RConn1 -- Bus_1/LConn2
  InPhaseC/RConn1 -- Bus_1/LConn3

== system Power_Grid_Fault_Analysis_2016/Bus_10 ==
  Bus Load 10 : powerlib/Elements/Three-Phase Series RLC Load  LConnTagsString=A|B|C  Configuration=Y (grounded)  NominalVoltage=basekV*1e3  Vabc=[1e3 1e3 1e3]  Vabcp=[1e3 1e3 1e3]  NominalFrequency=freq  UnbalancedPower=off  ActivePower=1e6  InductivePower=0.9e6  CapacitivePower=0  Pabc=[10e3 9e3 11e3]  QLabc=[100 90 110]  QCabc=[100 90 110]  Pabcp=[10e3 9e3 11e3]  QLabcp=[100 90 110]  QCabcp=[100 90 110]  Measurements=None  LoadType=constant PQ
  Bus_10 : powerlib/Measurements/Three-Phase V-I Measurement  VoltageMeasurement=phase-to-phase  SetLabelV=off  LabelV=Vabc  Vpu=off  VpuLL=off  CurrentMeasurement=yes  SetLabelI=off  LabelI=Iabc  Ipu=off  Pbase=100e6  Vbase=500e3  OutputType=Complex  PhasorSimulation=off  PSBequivalent=0
  VI Recorder7 : Subsystem
  InPhaseA : PMIOPort  Side=Left
  InPhaseB : PMIOPort  Port=2  Side=Left
  InPhaseC : PMIOPort  Port=3  Side=Left
  OutPhaseA : PMIOPort  Port=4  Side=Right
  OutPhaseB : PMIOPort  Port=5  Side=Right
  OutPhaseC : PMIOPort  Port=6  Side=Right
  wires:
  Bus_10/1 -> VI Recorder7/1(Vrec)
  Bus_10/2 -> VI Recorder7/2(Irec)
  connections:
  Bus Load 10/LConn1 -- OutPhaseA/RConn1 -- Bus_10/RConn1
  Bus_10/RConn2 -- OutPhaseB/RConn1 -- Bus Load 10/LConn2
  Bus Load 10/LConn3 -- OutPhaseC/RConn1 -- Bus_10/RConn3
  InPhaseA/RConn1 -- Bus_10/LConn1
  InPhaseB/RConn1 -- Bus_10/LConn2
  InPhaseC/RConn1 -- Bus_10/LConn3

== system Power_Grid_Fault_Analysis_2016/Bus_11 ==
  Bus Load 11 : powerlib/Elements/Three-Phase Series RLC Load  LConnTagsString=A|B|C  Configuration=Y (grounded)  NominalVoltage=basekV*1e3  Vabc=[1e3 1e3 1e3]  Vabcp=[1e3 1e3 1e3]  NominalFrequency=freq  UnbalancedPower=off  ActivePower=0.6e6  InductivePower=0.1e6  CapacitivePower=0.6e6  Pabc=[10e3 9e3 11e3]  QLabc=[100 90 110]  QCabc=[100 90 110]  Pabcp=[10e3 9e3 11e3]  QLabcp=[100 90 110]  QCabcp=[100 90 110]  Measurements=None  LoadType=constant PQ
  Bus_11 : powerlib/Measurements/Three-Phase V-I Measurement  VoltageMeasurement=phase-to-phase  SetLabelV=off  LabelV=Vabc  Vpu=off  VpuLL=off  CurrentMeasurement=yes  SetLabelI=off  LabelI=Iabc  Ipu=off  Pbase=100e6  Vbase=500e3  OutputType=Complex  PhasorSimulation=off  PSBequivalent=0
  VI Recorder7 : Subsystem
  InPhaseA : PMIOPort  Side=Left
  InPhaseB : PMIOPort  Port=2  Side=Left
  InPhaseC : PMIOPort  Port=3  Side=Left
  OutPhaseA : PMIOPort  Port=4  Side=Right
  OutPhaseB : PMIOPort  Port=5  Side=Right
  OutPhaseC : PMIOPort  Port=6  Side=Right
  wires:
  Bus_11/1 -> VI Recorder7/1(Vrec)
  Bus_11/2 -> VI Recorder7/2(Irec)
  connections:
  Bus Load 11/LConn1 -- OutPhaseA/RConn1 -- Bus_11/RConn1
  Bus_11/RConn2 -- OutPhaseB/RConn1 -- Bus Load 11/LConn2
  Bus Load 11/LConn3 -- OutPhaseC/RConn1 -- Bus_11/RConn3
  InPhaseA/RConn1 -- Bus_11/LConn1
  InPhaseB/RConn1 -- Bus_11/LConn2
  InPhaseC/RConn1 -- Bus_11/LConn3

== system Power_Grid_Fault_Analysis_2016/Bus_12 ==
  Bus Load 12 : powerlib/Elements/Three-Phase Series RLC Load  LConnTagsString=A|B|C  Configuration=Y (grounded)  NominalVoltage=basekV*1e3  Vabc=[1e3 1e3 1e3]  Vabcp=[1e3 1e3 1e3]  NominalFrequency=freq  UnbalancedPower=off  ActivePower=4.5e6  InductivePower=2.0e6  CapacitivePower=3.7e6  Pabc=[10e3 9e3 11e3]  QLabc=[100 90 110]  QCabc=[100 90 110]  Pabcp=[10e3 9e3 11e3]  QLabcp=[100 90 110]  QCabcp=[100 90 110]  Measurements=None  LoadType=constant PQ
  Bus_12 : powerlib/Measurements/Three-Phase V-I Measurement  VoltageMeasurement=phase-to-phase  SetLabelV=off  LabelV=Vabc  Vpu=off  VpuLL=off  CurrentMeasurement=yes  SetLabelI=off  LabelI=Iabc  Ipu=off  Pbase=100e6  Vbase=500e3  OutputType=Complex  PhasorSimulation=off  PSBequivalent=0
  VI Recorder7 : Subsystem
  InPhaseA : PMIOPort  Side=Left
  InPhaseB : PMIOPort  Port=2  Side=Left
  InPhaseC : PMIOPort  Port=3  Side=Left
  OutPhaseA : PMIOPort  Port=4  Side=Right
  OutPhaseB : PMIOPort  Port=5  Side=Right
  OutPhaseC : PMIOPort  Port=6  Side=Right
  wires:
  Bus_12/1 -> VI Recorder7/1(Vrec)
  Bus_12/2 -> VI Recorder7/2(Irec)
  connections:
  Bus Load 12/LConn1 -- OutPhaseA/RConn1 -- Bus_12/RConn1
  Bus_12/RConn2 -- OutPhaseB/RConn1 -- Bus Load 12/LConn2
  Bus Load 12/LConn3 -- OutPhaseC/RConn1 -- Bus_12/RConn3
  InPhaseA/RConn1 -- Bus_12/LConn1
  InPhaseB/RConn1 -- Bus_12/LConn2
  InPhaseC/RConn1 -- Bus_12/LConn3

== system Power_Grid_Fault_Analysis_2016/Bus_13 ==
  Bus Load 13 : powerlib/Elements/Three-Phase Series RLC Load  LConnTagsString=A|B|C  Configuration=Y (grounded)  NominalVoltage=basekV*1e3  Vabc=[1e3 1e3 1e3]  Vabcp=[1e3 1e3 1e3]  NominalFrequency=freq  UnbalancedPower=off  ActivePower=1e6  InductivePower=0.9e6  CapacitivePower=0  Pabc=[10e3 9e3 11e3]  QLabc=[100 90 110]  QCabc=[100 90 110]  Pabcp=[10e3 9e3 11e3]  QLabcp=[100 90 110]  QCabcp=[100 90 110]  Measurements=None  LoadType=constant PQ
  Bus_13 : powerlib/Measurements/Three-Phase V-I Measurement  VoltageMeasurement=phase-to-phase  SetLabelV=off  LabelV=Vabc  Vpu=off  VpuLL=off  CurrentMeasurement=yes  SetLabelI=off  LabelI=Iabc  Ipu=off  Pbase=100e6  Vbase=500e3  OutputType=Complex  PhasorSimulation=off  PSBequivalent=0
  VI Recorder7 : Subsystem
  InPhaseA : PMIOPort  Side=Left
  InPhaseB : PMIOPort  Port=2  Side=Left
  InPhaseC : PMIOPort  Port=3  Side=Left
  OutPhaseA : PMIOPort  Port=4  Side=Right
  OutPhaseB : PMIOPort  Port=5  Side=Right
  OutPhaseC : PMIOPort  Port=6  Side=Right
  wires:
  Bus_13/1 -> VI Recorder7/1(Vrec)
  Bus_13/2 -> VI Recorder7/2(Irec)
  connections:
  Bus Load 13/LConn1 -- OutPhaseA/RConn1 -- Bus_13/RConn1
  Bus_13/RConn2 -- OutPhaseB/RConn1 -- Bus Load 13/LConn2
  Bus Load 13/LConn3 -- OutPhaseC/RConn1 -- Bus_13/RConn3
  InPhaseA/RConn1 -- Bus_13/LConn1
  InPhaseB/RConn1 -- Bus_13/LConn2
  InPhaseC/RConn1 -- Bus_13/LConn3

== system Power_Grid_Fault_Analysis_2016/Bus_14 ==
  Bus Load 14 : powerlib/Elements/Three-Phase Series RLC Load  LConnTagsString=A|B|C  Configuration=Y (grounded)  NominalVoltage=basekV*1e3  Vabc=[1e3 1e3 1e3]  Vabcp=[1e3 1e3 1e3]  NominalFrequency=freq  UnbalancedPower=off  ActivePower=1e6  InductivePower=0.7e6  CapacitivePower=1.8e6  Pabc=[10e3 9e3 11e3]  QLabc=[100 90 110]  QCabc=[100 90 110]  Pabcp=[10e3 9e3 11e3]  QLabcp=[100 90 110]  QCabcp=[100 90 110]  Measurements=None  LoadType=constant PQ
  Bus_14 : powerlib/Measurements/Three-Phase V-I Measurement  VoltageMeasurement=phase-to-phase  SetLabelV=off  LabelV=Vabc  Vpu=off  VpuLL=off  CurrentMeasurement=yes  SetLabelI=off  LabelI=Iabc  Ipu=off  Pbase=100e6  Vbase=500e3  OutputType=Complex  PhasorSimulation=off  PSBequivalent=0
  VI Recorder7 : Subsystem
  InPhaseA : PMIOPort  Side=Left
  InPhaseB : PMIOPort  Port=2  Side=Left
  InPhaseC : PMIOPort  Port=3  Side=Left
  OutPhaseA : PMIOPort  Port=4  Side=Right
  OutPhaseB : PMIOPort  Port=5  Side=Right
  OutPhaseC : PMIOPort  Port=6  Side=Right
  wires:
  Bus_14/1 -> VI Recorder7/1(Vrec)
  Bus_14/2 -> VI Recorder7/2(Irec)
  connections:
  Bus Load 14/LConn1 -- OutPhaseA/RConn1 -- Bus_14/RConn1
  Bus_14/RConn2 -- OutPhaseB/RConn1 -- Bus Load 14/LConn2
  Bus Load 14/LConn3 -- OutPhaseC/RConn1 -- Bus_14/RConn3
  InPhaseA/RConn1 -- Bus_14/LConn1
  InPhaseB/RConn1 -- Bus_14/LConn2
  InPhaseC/RConn1 -- Bus_14/LConn3

== system Power_Grid_Fault_Analysis_2016/Bus_15 ==
  Bus Load 15 : powerlib/Elements/Three-Phase Series RLC Load  LConnTagsString=A|B|C  Configuration=Y (grounded)  NominalVoltage=basekV*1e3  Vabc=[1e3 1e3 1e3]  Vabcp=[1e3 1e3 1e3]  NominalFrequency=freq  UnbalancedPower=off  ActivePower=1e6  InductivePower=0.9e6  CapacitivePower=0  Pabc=[10e3 9e3 11e3]  QLabc=[100 90 110]  QCabc=[100 90 110]  Pabcp=[10e3 9e3 11e3]  QLabcp=[100 90 110]  QCabcp=[100 90 110]  Measurements=None  LoadType=constant PQ
  Bus_15 : powerlib/Measurements/Three-Phase V-I Measurement  VoltageMeasurement=phase-to-phase  SetLabelV=off  LabelV=Vabc  Vpu=off  VpuLL=off  CurrentMeasurement=yes  SetLabelI=off  LabelI=Iabc  Ipu=off  Pbase=100e6  Vbase=500e3  OutputType=Complex  PhasorSimulation=off  PSBequivalent=0
  VI Recorder7 : Subsystem
  InPhaseA : PMIOPort  Side=Left
  InPhaseB : PMIOPort  Port=2  Side=Left
  InPhaseC : PMIOPort  Port=3  Side=Left
  OutPhaseA : PMIOPort  Port=4  Side=Right
  OutPhaseB : PMIOPort  Port=5  Side=Right
  OutPhaseC : PMIOPort  Port=6  Side=Right
  wires:
  Bus_15/1 -> VI Recorder7/1(Vrec)
  Bus_15/2 -> VI Recorder7/2(Irec)
  connections:
  Bus Load 15/LConn1 -- OutPhaseA/RConn1 -- Bus_15/RConn1
  Bus_15/RConn2 -- OutPhaseB/RConn1 -- Bus Load 15/LConn2
  Bus Load 15/LConn3 -- OutPhaseC/RConn1 -- Bus_15/RConn3
  InPhaseA/RConn1 -- Bus_15/LConn1
  InPhaseB/RConn1 -- Bus_15/LConn2
  InPhaseC/RConn1 -- Bus_15/LConn3

== system Power_Grid_Fault_Analysis_2016/Bus_16 ==
  Bus Load 16 : powerlib/Elements/Three-Phase Series RLC Load  LConnTagsString=A|B|C  Configuration=Y (grounded)  NominalVoltage=basekV*1e3  Vabc=[1e3 1e3 1e3]  Vabcp=[1e3 1e3 1e3]  NominalFrequency=freq  UnbalancedPower=off  ActivePower=2.1e6  InductivePower=1.0e6  CapacitivePower=1.8e6  Pabc=[10e3 9e3 11e3]  QLabc=[100 90 110]  QCabc=[100 90 110]  Pabcp=[10e3 9e3 11e3]  QLabcp=[100 90 110]  QCabcp=[100 90 110]  Measurements=None  LoadType=constant PQ
  Bus_16 : powerlib/Measurements/Three-Phase V-I Measurement  VoltageMeasurement=phase-to-phase  SetLabelV=off  LabelV=Vabc  Vpu=off  VpuLL=off  CurrentMeasurement=yes  SetLabelI=off  LabelI=Iabc  Ipu=off  Pbase=100e6  Vbase=500e3  OutputType=Complex  PhasorSimulation=off  PSBequivalent=0
  VI Recorder7 : Subsystem
  InPhaseA : PMIOPort  Side=Left
  InPhaseB : PMIOPort  Port=2  Side=Left
  InPhaseC : PMIOPort  Port=3  Side=Left
  OutPhaseA : PMIOPort  Port=4  Side=Right
  OutPhaseB : PMIOPort  Port=5  Side=Right
  OutPhaseC : PMIOPort  Port=6  Side=Right
  wires:
  Bus_16/1 -> VI Recorder7/1(Vrec)
  Bus_16/2 -> VI Recorder7/2(Irec)
  connections:
  Bus Load 16/LConn1 -- OutPhaseA/RConn1 -- Bus_16/RConn1
  Bus_16/RConn2 -- OutPhaseB/RConn1 -- Bus Load 16/LConn2
  Bus Load 16/LConn3 -- OutPhaseC/RConn1 -- Bus_16/RConn3
  InPhaseA/RConn1 -- Bus_16/LConn1
  InPhaseB/RConn1 -- Bus_16/LConn2
  InPhaseC/RConn1 -- Bus_16/LConn3
